simulink model "s10_9"  (Simulink 6.6)
settings: Solver=ode45  SolverMode=SingleTasking  StartTime=0.0  StopTime=t_d  MaxStep=Tc  RelTol=1e-6  AbsTol=1e-6
values from neighbouring files (symbols this model uses):
  K = eye(4)    [i10_9.m]
  k_s = 160    [i10_9.m]
  q_i = inv_ksu(a,x_i)    [i10_9.m]
  Tc = 0.04    [i10_9.m]
  Te = 0.001    [i10_9.m]
  Ts = Tc    (= 0.04)    [i10_9.m]
  x_do = [-0.1; 0.1; 0.6; -pi/3]    [i10_9.m]
  x_o = [1; 1; 1; pi/4]    [i10_9.m]
  xh0 = x_do    [i10_9.m]
undefined symbols (not defined in the file or in its folder): a, DiscIntNeverNeededParam
settings Model: Creator=luigivillani  LastModifiedBy=luigivillani  ExtModeAutoUpdateStatusClock=off
settings DataIOCC: LimitDataPoints=off  SaveOutput=off  SaveTime=off  SignalLoggingName=sigsOut
settings OptimizationCC: BooleanDataType=off
settings DebuggingCC: SignalResolutionControl=TryResolveAllWithWarning  SolverPrmCheckMsg=none  MultiTaskDSMMsg=warning  MultiTaskCondExecSysMsg=none  StrictBusMsg=None
settings HardwareCC: TargetUnknown=on
settings RTWCC: IncludeERTFirstTime=on

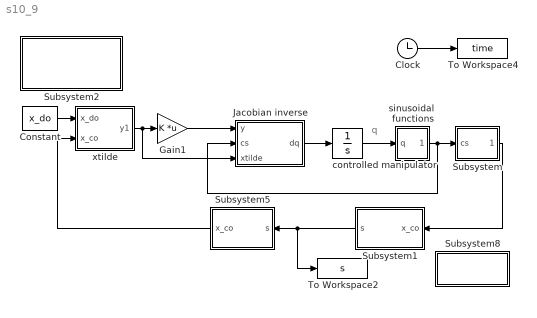
== system s10_9 ==
  note: q
  Clock : Clock
      settings: Decimation=10
  Constant : Constant  Value=x_do  SampleTime=Tc
  Gain1 : Gain  Gain=K  Multiplication=Matrix(K*u)  SampleTime=Tc
      mask Display: disp('K')
  Jacobian inverse : Subsystem
      mask Display: disp('inv(J_Aq(q))')
  Subsystem : Subsystem
  Subsystem1 : Subsystem  Orientation=left
      mask Display: disp('features')
  Subsystem2 : Subsystem
      settings: OpenFcn=clear all;i10_9;
      mask Display: disp('variables\n initialization')
  Subsystem5 : Subsystem  Orientation=left
      mask Display: disp('estimate')
  Subsystem8 : Subsystem
      settings: OpenFcn=p10_9;
      mask Display: disp('plot')
  To Workspace2 : ToWorkspace  VariableName=s  SampleTime=Ts  SaveFormat=Array
      settings: MaxDataPoints=4001
  To Workspace4 : ToWorkspace  VariableName=time  SampleTime=Ts  SaveFormat=Array
      settings: MaxDataPoints=4001
  controlled manipulator : Integrator  InitialCondition=q_i
  sinusoidal  functions : Subsystem
      mask Display: disp('cs(q)')
  xtilde : Subsystem
      mask Display: disp('xtilde')
  wires:
  Clock/1 -> To Workspace4/1
  Constant/1 -> xtilde/1(x_do)
  controlled manipulator/1 -> sinusoidal  functions/1(q)
  xtilde/1(y1) -> Gain1/1, Jacobian inverse/3(xtilde)
  Subsystem5/1(x_co) -> xtilde/2(x_co)
  sinusoidal  functions/1(cs) -> Subsystem/1(cs), Jacobian inverse/2(cs)
  Subsystem1/1(s) -> Subsystem5/1(s), To Workspace2/1
  Subsystem/1(x_co) -> Subsystem1/1(x_co)
  Gain1/1 -> Jacobian inverse/1(y)
  Jacobian inverse/1(dq) -> controlled manipulator/1

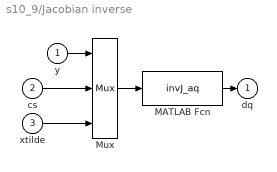
== system s10_9/Jacobian inverse ==
  y : Inport
  cs : Inport  Port=2
  xtilde : Inport  Port=3
  MATLAB Fcn : MATLABFcn  MATLABFcn=invJ_aq  OutputDimensions=4  SampleTime=Tc
      mask Display: disp('inv(J_Aq(q))y')
  Mux : Mux  Inputs=[4,6,4]
  dq : Outport  InitialOutput=0
  wires:
  MATLAB Fcn/1 -> dq/1
  Mux/1 -> MATLAB Fcn/1
  cs/1 -> Mux/2
  y/1 -> Mux/1
  xtilde/1 -> Mux/3

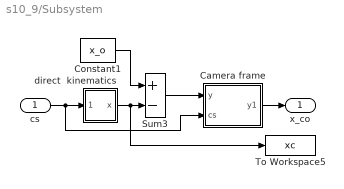
== system s10_9/Subsystem ==
  cs : Inport
  Camera frame : Subsystem
      mask Display: disp('c_frame')
  Constant1 : Constant  Value=x_o  SampleTime=Tc
  Sum3 : Sum  Inputs=+-  SaturateOnIntegerOverflow=on  InputSameDT=on
  To Workspace5 : ToWorkspace  VariableName=xc  SampleTime=Ts  SaveFormat=Array
      settings: MaxDataPoints=4001
  direct  kinematics : Subsystem
      mask Display: disp('k(q)')
  x_co : Outport
  wires:
  Constant1/1 -> Sum3/1
  direct  kinematics/1(x) -> To Workspace5/1, Sum3/2
  Sum3/1 -> Camera frame/1(y)
  cs/1 -> direct  kinematics/1(cs), Camera frame/2(cs)
  Camera frame/1(y1) -> x_co/1

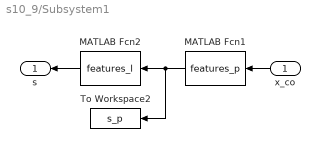
== system s10_9/Subsystem1 ==
  x_co : Inport  Orientation=left
  MATLAB Fcn1 : MATLABFcn  Orientation=left  MATLABFcn=features_p  OutputDimensions=4  SampleTime=Tc
      mask Display: disp('points')
  MATLAB Fcn2 : MATLABFcn  Orientation=left  MATLABFcn=features_l  OutputDimensions=4
      mask Display: disp('line')
  To Workspace2 : ToWorkspace  VariableName=s_p  SampleTime=Ts  SaveFormat=Array
      settings: MaxDataPoints=4001
  s : Outport  Orientation=left
  wires:
  MATLAB Fcn1/1 -> MATLAB Fcn2/1, To Workspace2/1
  x_co/1 -> MATLAB Fcn1/1
  MATLAB Fcn2/1 -> s/1

== system s10_9/Subsystem2 ==
  note: start

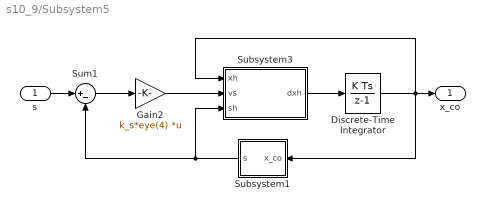
== system s10_9/Subsystem5 ==
  s : Inport
  Discrete-Time Integrator : DiscreteIntegrator  InitialCondition=xh0  SampleTime=Te  ICPrevOutput=DiscIntNeverNeededParam  ICPrevScaledInput=DiscIntNeverNeededParam
  Gain2 : Gain  Gain=k_s*eye(4)  Multiplication=Matrix(K*u)  SampleTime=Te
      mask Display: disp('K_s')
  Subsystem1 : Subsystem  Orientation=left
      mask Display: disp('s(xh)')
  Subsystem3 : Subsystem
      mask Display: disp('inv(J_asl)vs')
  Sum1 : Sum  Inputs=|+-  SampleTime=Te  SaturateOnIntegerOverflow=on
  x_co : Outport
  wires:
  Discrete-Time Integrator/1 -> Subsystem3/1(xh), x_co/1, Subsystem1/1(x_co)
  Subsystem3/1(dxh) -> Discrete-Time Integrator/1
  Gain2/1 -> Subsystem3/2(vs)
  Subsystem1/1(s) -> Sum1/2, Subsystem3/3(sh)
  Sum1/1 -> Gain2/1
  s/1 -> Sum1/1

== system s10_9/Subsystem8 ==
  note: start

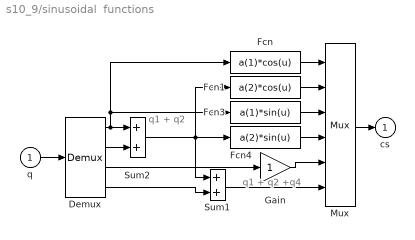
== system s10_9/sinusoidal  functions ==
  note: q1 + q2
  note: q1 + q2 +q4
  q : Inport
  Demux : Demux
  Fcn : Fcn  Expr=a(1)*cos(u)  SampleTime=Tc
  Fcn1 : Fcn  Expr=a(2)*cos(u)  SampleTime=Tc
  Fcn3 : Fcn  Expr=a(1)*sin(u)  SampleTime=Tc
  Fcn4 : Fcn  Expr=a(2)*sin(u)  SampleTime=Tc
  Gain : Gain  SampleTime=Tc
  Mux : Mux  Inputs=6
  Sum1 : Sum  SampleTime=Tc  SaturateOnIntegerOverflow=on  InputSameDT=on
  Sum2 : Sum  SampleTime=Tc  SaturateOnIntegerOverflow=on  InputSameDT=on
  cs : Outport  InitialOutput=0
  wires:
  Fcn/1 -> Mux/1
  Mux/1 -> cs/1
  Demux/2 -> Sum2/2
  Sum2/1 -> Fcn1/1, Fcn4/1, Sum1/1
  Demux/1 -> Sum2/1, Fcn/1, Fcn3/1
  Fcn1/1 -> Mux/2
  Fcn3/1 -> Mux/3
  Fcn4/1 -> Mux/4
  q/1 -> Demux/1
  Demux/4 -> Sum1/2
  Sum1/1 -> Mux/6
  Demux/3 -> Gain/1
  Gain/1 -> Mux/5

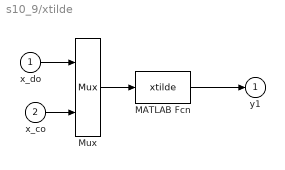
== system s10_9/xtilde ==
  x_do : Inport
  x_co : Inport  Port=2
  MATLAB Fcn : MATLABFcn  MATLABFcn=xtilde  OutputDimensions=4  SampleTime=Tc
      mask Display: disp('xtilde')
  Mux : Mux  Inputs=[4,4]
  y1 : Outport  InitialOutput=0
  wires:
  MATLAB Fcn/1 -> y1/1
  Mux/1 -> MATLAB Fcn/1
  x_co/1 -> Mux/2
  x_do/1 -> Mux/1

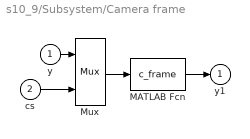
== system s10_9/Subsystem/Camera frame ==
  y : Inport
  cs : Inport  Port=2
  MATLAB Fcn : MATLABFcn  MATLABFcn=c_frame  OutputDimensions=4
      mask Display: disp('c_frame')
  Mux : Mux  Inputs=[4,6]
  y1 : Outport  InitialOutput=0
  wires:
  MATLAB Fcn/1 -> y1/1
  Mux/1 -> MATLAB Fcn/1
  y/1 -> Mux/1
  cs/1 -> Mux/2

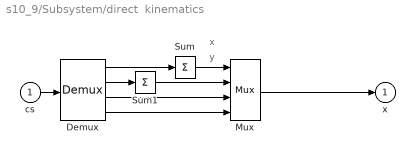
== system s10_9/Subsystem/direct  kinematics ==
  note: y
  note: x
  cs : Inport
  Demux : Demux  Outputs=[2,2,1,1]
  Mux : Mux
  Sum : Sum  Inputs=+  SaturateOnIntegerOverflow=on  InputSameDT=on
  Sum1 : Sum  Inputs=+  SaturateOnIntegerOverflow=on  InputSameDT=on
  x : Outport  InitialOutput=0
  wires:
  Sum1/1 -> Mux/2
  Sum/1 -> Mux/1
  Demux/2 -> Sum1/1
  Demux/1 -> Sum/1
  cs/1 -> Demux/1
  Mux/1 -> x/1
  Demux/4 -> Mux/4
  Demux/3 -> Mux/3

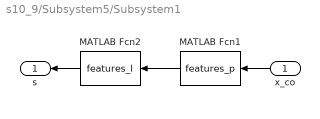
== system s10_9/Subsystem5/Subsystem1 ==
  x_co : Inport  Orientation=left
  MATLAB Fcn1 : MATLABFcn  Orientation=left  MATLABFcn=features_p  OutputDimensions=4  SampleTime=Te
      mask Display: disp('points')
  MATLAB Fcn2 : MATLABFcn  Orientation=left  MATLABFcn=features_l  OutputDimensions=4  SampleTime=Te
      mask Display: disp('line')
  s : Outport  Orientation=left
  wires:
  MATLAB Fcn1/1 -> MATLAB Fcn2/1
  x_co/1 -> MATLAB Fcn1/1
  MATLAB Fcn2/1 -> s/1

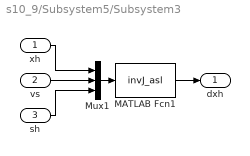
== system s10_9/Subsystem5/Subsystem3 ==
  xh : Inport
  vs : Inport  Port=2
  sh : Inport  Port=3
  MATLAB Fcn1 : MATLABFcn  MATLABFcn=invJ_asl  OutputDimensions=4  SampleTime=Te
      mask Display: disp('inv(J_asl)')
  Mux1 : Mux  Inputs=[4,4,4]
  dxh : Outport
  wires:
  Mux1/1 -> MATLAB Fcn1/1
  xh/1 -> Mux1/1
  sh/1 -> Mux1/3
  MATLAB Fcn1/1 -> dxh/1
  vs/1 -> Mux1/2
